simulink subsystem "Sub_Motores"  (R2023b)
settings: Solver=VariableStepAuto  StartTime=0.0  StopTime=10.0  RelTol=1e-3
libraries: arduinolib x6, simulink x2
settings Model: Creator=Usuario  LastModifiedBy=Usuario

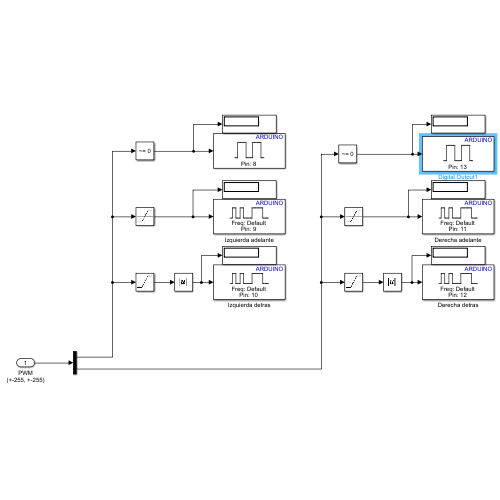
[thumbnail: Simulink's stored preview of the top-level diagram]
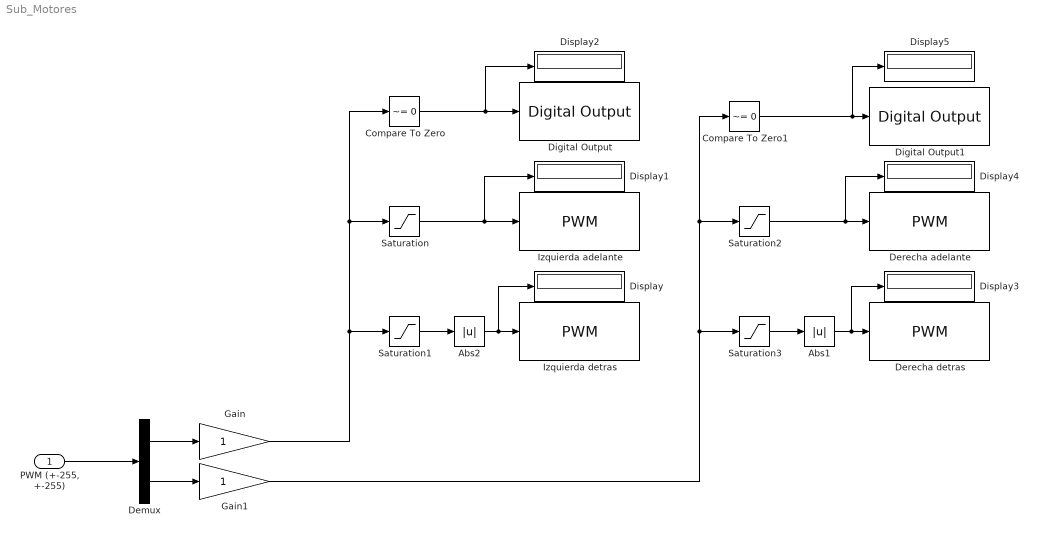
== system Sub_Motores ==
  "PWM (+-255, +-255)" : Inport
  Abs1 : Abs  SaturateOnIntegerOverflow=off
  Abs2 : Abs  SaturateOnIntegerOverflow=off
  Compare To Zero : simulink/Logic and Bit Operations/Compare To Zero  relop=~=  OutDataTypeStr=boolean
  Compare To Zero1 : simulink/Logic and Bit Operations/Compare To Zero  relop=~=  OutDataTypeStr=boolean
  Demux : Demux  Outputs=2
  Derecha adelante : arduinolib/PWM  pinNumber=10  frequencyType=Default  desiredFrequency=490.2  achievableFrequency=490.2
  Derecha detras : arduinolib/PWM  pinNumber=9  frequencyType=Default  desiredFrequency=490.2  achievableFrequency=490.2
  Digital Output : arduinolib/Digital Output  pinNumber=13  Direction=output  blockPlatform=arduino
  Digital Output1 : arduinolib/Digital Output  pinNumber=8  Direction=output  blockPlatform=arduino
  Display{,1..5} (6 alike) : Display
  Gain : Gain
  Gain1 : Gain
  Izquierda adelante : arduinolib/PWM  pinNumber=12  frequencyType=Default  desiredFrequency=490.2  achievableFrequency=490.2
  Izquierda detras : arduinolib/PWM  pinNumber=11  frequencyType=Default  desiredFrequency=490.2  achievableFrequency=490.2
  Saturation : Saturate  UpperLimit=255  LowerLimit=0
  Saturation1 : Saturate  UpperLimit=0  LowerLimit=-255
  Saturation2 : Saturate  UpperLimit=255  LowerLimit=0
  Saturation3 : Saturate  UpperLimit=0  LowerLimit=-255
  wires:
  Abs2/1 -> Izquierda detras/1, Display/1
  Demux/1 -> Gain/1
  Abs1/1 -> Derecha detras/1, Display3/1
  Saturation/1 -> Izquierda adelante/1, Display1/1
  Saturation1/1 -> Abs2/1
  Saturation2/1 -> Derecha adelante/1, Display4/1
  Compare To Zero1/1 -> Display5/1, Digital Output1/1
  Compare To Zero/1 -> Digital Output/1, Display2/1
  Saturation3/1 -> Abs1/1
  "PWM (+-255, +-255)"/1 -> Demux/1
  Demux/2 -> Gain1/1
  Gain/1 -> Compare To Zero/1, Saturation/1, Saturation1/1
  Gain1/1 -> Saturation3/1, Compare To Zero1/1, Saturation2/1
